simulink model "test3_px4"  (R2022b)
settings: Solver=ode4  StartTime=0.0  StopTime=inf  FixedStep=0.004  RelTol=1e-3
undefined symbols (not defined in the file or in its folder): Earth, WGS84
libraries: shared6dof x1, aerolibatmos2 x1, aerolibtransform2 x1, test_px4 x1
settings Model: PauseTimes=30  Creator=User  LastModifiedBy=User

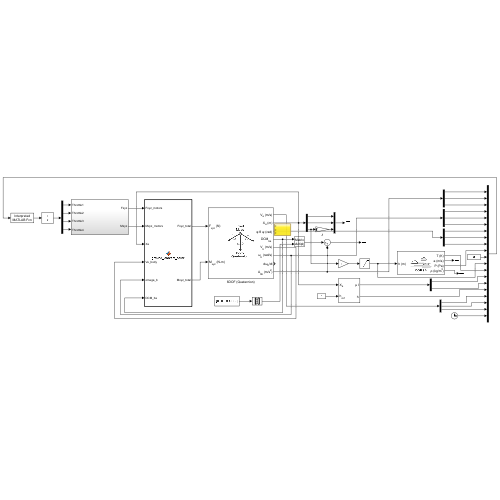
[thumbnail: Simulink's stored preview of the top-level diagram]
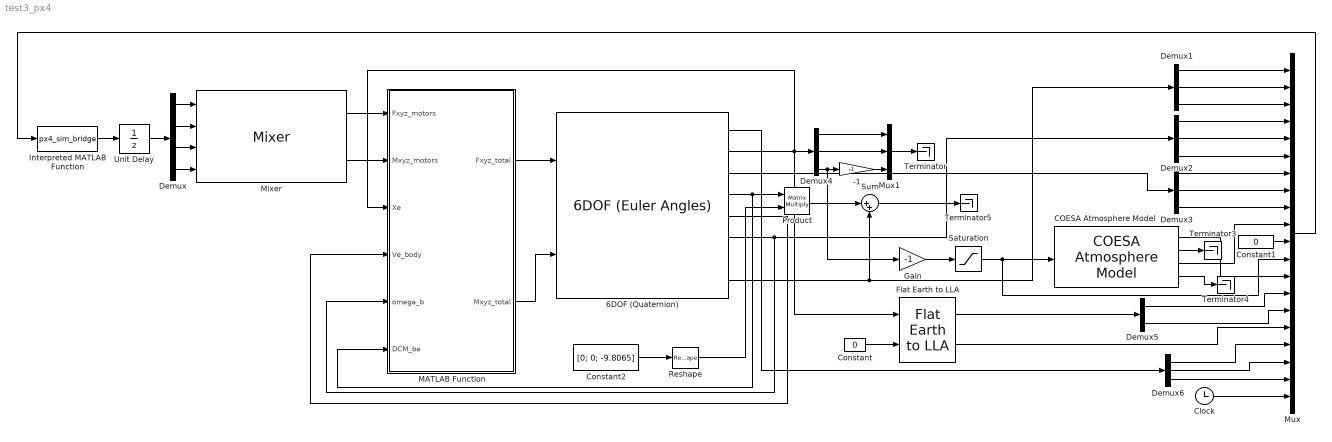
== system test3_px4 ==
  -1 : Gain  Gain=-1
  6DOF (Quaternion) : shared6dof/6DOF (Euler Angles)  units=Metric (MKS)  mtype=Fixed  rep=Quaternion  xme_0=[0 0 0]  Vm_0=[0 0 0]  eul_0=[0 0 0]  pm_0=[0 0 0]  mass_0=1.0  mass_e=0.5  mass_f=2.0  inertia=eye(3)  inertia_e=eye(3)  inertia_f=2*eye(3)  k_quat=1.0  vre_flag=on  abi_flag=off  aMode=0  xme_statename=''  Vm_statename=''  eul_statename=''  quat_statename=''  pm_statename=''  mass_statename=''
      settings: LibrarySourceBlock=aerolib6dof2/6DOF (Quaternion)
  COESA Atmosphere Model : aerolibatmos2/COESA Atmosphere Model  units=Metric (MKS)  spec=1976 COESA-extended U.S. Standard Atmosphere  model=Profile  profile_var=High temperature  profile_percent=1%  profile_alt=5 km (16404 ft)  envelope_var=High temperature  envelope_percent=1%  action=Warning
  Clock : Clock
  Constant : Constant  Value=0
  Constant1 : Constant  Value=0
  Constant2 : Constant  Value=[0; 0; -9.8065]
  Demux : Demux
  Demux{1..4,6} (5 alike) : Demux  Outputs=3
  Demux5 : Demux  Outputs=2
  Flat Earth to LLA : aerolibtransform2/Flat Earth to LLA  units=Metric (MKS)  ptype=Earth (WGS84)  F=1/298.257223563  R=6378137  refPosPort=off  LL0=[0 10]  psi=0
  Gain : Gain  Gain=-1
  Interpreted MATLAB Function : MATLABFcn  MATLABFcn=px4_sim_bridge  OutputDimensions=4  OutputSignalType=real
  MATLAB Function : MATLAB Function  TreatAsAtomicUnit=on
  Mixer : test_px4/Mixer  SystemSampleTime=-1  VariantActivationTime=update diagram  Latency=0  AutoFrameSizeCalculation=off
  Mux : Mux  Inputs=20
  Mux1 : Mux  Inputs=3
  Product : Product  Multiplication=Matrix(*)
  Reshape : Reshape  OutputDimensionality=Column vector (2-D)
  Saturation : Saturate  UpperLimit=84852  LowerLimit=0
  Sum : Sum  Inputs=|++
  Terminator{,3..5} (4 alike) : Terminator
  Unit Delay : UnitDelay  SampleTime=0.004  HasFrameUpgradeWarning=on
  wires:
  6DOF (Quaternion)/6 -> Demux2/1, MATLAB Function/5(omega_b)
  6DOF (Quaternion)/8 -> Demux1/1, Sum/2
  Demux/3 -> Mixer/3
  Demux/1 -> Mixer/1
  MATLAB Function/1(Fxyz_total) -> 6DOF (Quaternion)/1
  Interpreted MATLAB Function/1 -> Unit Delay/1
  Unit Delay/1 -> Demux/1
  MATLAB Function/2(Mxyz_total) -> 6DOF (Quaternion)/2
  Demux/4 -> Mixer/4
  Demux/2 -> Mixer/2
  Demux1/1 -> Mux/1
  Demux1/2 -> Mux/2
  Demux1/3 -> Mux/3
  Demux2/1 -> Mux/4
  Demux2/2 -> Mux/5
  Demux2/3 -> Mux/6
  6DOF (Quaternion)/3 -> Demux3/1
  Demux3/1 -> Mux/7
  Demux3/2 -> Mux/8
  Demux3/3 -> Mux/9
  6DOF (Quaternion)/2 -> MATLAB Function/3(Xe), Flat Earth to LLA/1, Demux4/1
  Gain/1 -> Saturation/1
  Demux4/3 -> Gain/1, -1/1
  Constant/1 -> Flat Earth to LLA/2
  Flat Earth to LLA/1 -> Demux5/1
  COESA Atmosphere Model/3 -> Mux/10
  Constant1/1 -> Mux/11
  COESA Atmosphere Model/1 -> Mux/13
  Demux5/1 -> Mux/14
  Demux5/2 -> Mux/15
  Flat Earth to LLA/2 -> Mux/16
  6DOF (Quaternion)/1 -> Demux6/1
  Demux6/1 -> Mux/17
  Demux6/2 -> Mux/18
  Demux6/3 -> Mux/19
  Clock/1 -> Mux/20
  Mux/1 -> Interpreted MATLAB Function/1
  Demux4/1 -> Mux1/1
  Demux4/2 -> Mux1/2
  6DOF (Quaternion)/4 -> MATLAB Function/6(DCM_be), Product/1
  Constant2/1 -> Reshape/1
  Product/1 -> Sum/1
  COESA Atmosphere Model/2 -> Terminator3/1
  COESA Atmosphere Model/4 -> Terminator4/1
  Sum/1 -> Terminator5/1
  Reshape/1 -> Product/2
  Saturation/1 -> COESA Atmosphere Model/1, Mux/12
  -1/1 -> Mux1/3
  Mixer/1 -> MATLAB Function/1(Fxyz_motors)
  Mixer/2 -> MATLAB Function/2(Mxyz_motors)
  6DOF (Quaternion)/5 -> MATLAB Function/4(Ve_body)
  Mux1/1 -> Terminator/1

== matlab function test3_px4/MATLAB Function ==
  data: Fxyz_motors input; Fxyz_total output; Mxyz_motors input; Xe input; Ve_body input; omega_b input; DCM_be input; Mxyz_total output
function [Fxyz_total, Mxyz_total] = ground_contact_force(Fxyz_motors, Mxyz_motors, Xe, Ve_body, omega_b, DCM_be)
    [Fxyz_total, Mxyz_total] = ground_contact(Fxyz_motors, Mxyz_motors, Xe, Ve_body, omega_b, DCM_be);
